simulink model "Problema_a"  (R2023b)
settings: Solver=VariableStepAuto  StartTime=0.0  StopTime=10.0  RelTol=1e-3
settings Model: Creator=porti  LastModifiedBy=porti

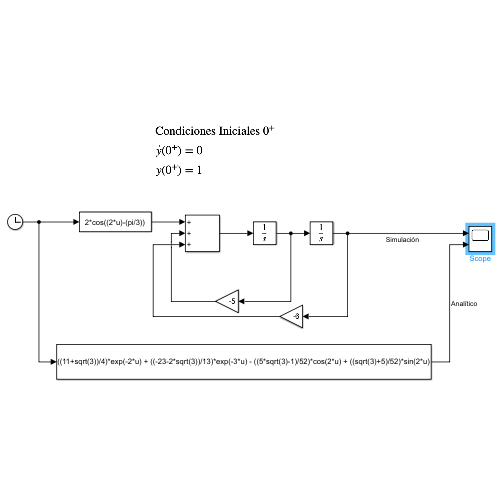
[thumbnail: Simulink's stored preview of the top-level diagram]
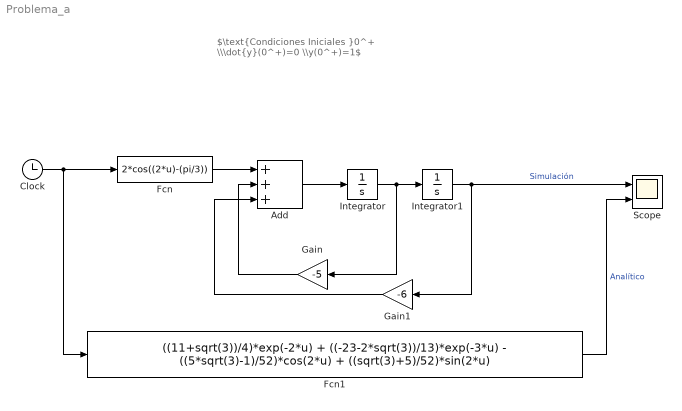
== system Problema_a ==
  note: $\text{Condiciones Iniciales }0^+ \\\dot{y}(0^+)=0 \\y(0^+)=1$
  Add : Sum  Inputs=+++
  Clock : Clock
  Fcn : Fcn  Expr=2*cos((2*u)-(pi/3))
  Fcn1 : Fcn  Expr=((11+sqrt(3))/4)*exp(-2*u) + ((-23-2*sqrt(3))/13)*exp(-3*u) - ((5*sqrt(3)-1)/52)*cos(2*u) + ((sqrt(3)+5)/52)*sin(2*u)
  Gain : Gain  Gain=-5
  Gain1 : Gain  Gain=-6
  Integrator : Integrator
  Integrator1 : Integrator  InitialCondition=1
  Scope : Scope  NumInputPorts=2
  wires:
  Fcn/1 -> Add/1
  Gain/1 -> Add/2
  Add/1 -> Integrator/1
  Integrator/1 -> Integrator1/1, Gain/1
  Integrator1/1 -> Gain1/1, Scope/1  "Simulación"
  Gain1/1 -> Add/3
  Clock/1 -> Fcn/1, Fcn1/1
  Fcn1/1 -> Scope/2  "Analítico"
